simulink library "csu_lat_landing_approach_targeting_lib"  (R2014b)
settings: Solver=ode45  StartTime=0.0  StopTime=10.0  RelTol=1e-3
libraries: simulink x8, util_info_lib x1, util_common_lib x1
settings Model: Creator=escrane  LastModifiedBy=Mark Agbayani

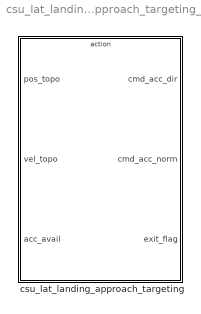
== system csu_lat_landing_approach_targeting_lib ==
  csu_lat_landing_approach_targeting : Subsystem  TreatAsAtomicUnit=on

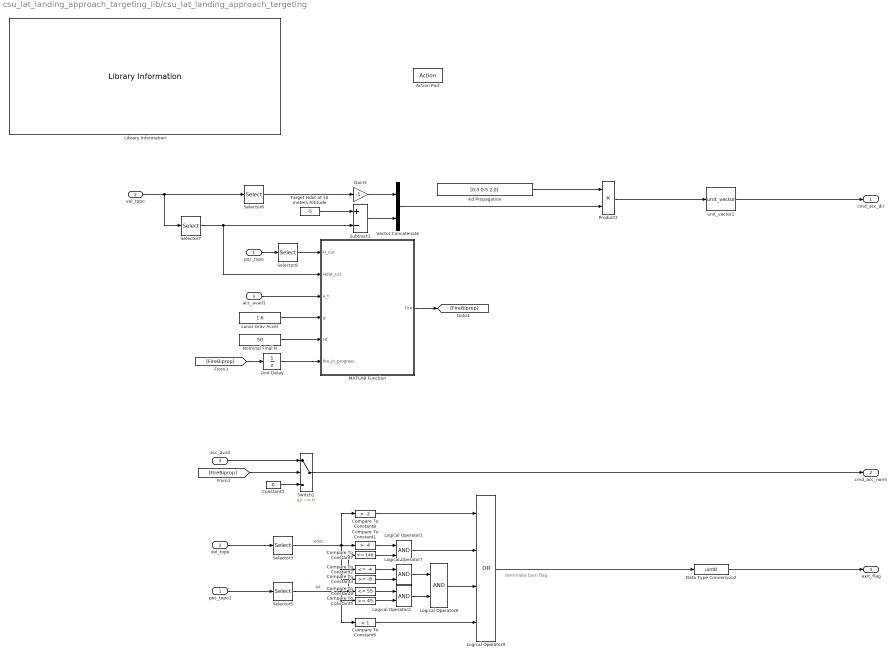
== system csu_lat_landing_approach_targeting_lib/csu_lat_landing_approach_targeting ==
  note: terminate burn flag
  "pos_topo " : Inport
  "vel_topo " : Inport  Port=2
  acc_avail : Inport  Port=3
  Action Port : ActionPort
  Compare To Constant1 : simulink/Logic and Bit Operations/Compare To Constant  relop=>  const=-4  OutDataTypeStr=boolean
  Compare To Constant2 : simulink/Logic and Bit Operations/Compare To Constant  relop=<=  const=-4  OutDataTypeStr=boolean
  Compare To Constant3 : simulink/Logic and Bit Operations/Compare To Constant  relop=>=  const=-8  OutDataTypeStr=boolean
  Compare To Constant4 : simulink/Logic and Bit Operations/Compare To Constant  relop=<=  const=55  OutDataTypeStr=boolean
  Compare To Constant5 : simulink/Logic and Bit Operations/Compare To Constant  relop=>=  const=45  OutDataTypeStr=boolean
  Compare To Constant6 : simulink/Logic and Bit Operations/Compare To Constant  relop=<  const=1  OutDataTypeStr=boolean
  Compare To Constant7 : simulink/Logic and Bit Operations/Compare To Constant  relop=<=  const=140  OutDataTypeStr=boolean
  Compare To Constant8 : simulink/Logic and Bit Operations/Compare To Constant  relop=>  const=-2  OutDataTypeStr=boolean
  Constant3 : Constant  Value=0
  Data Type Conversion2 : DataTypeConversion  OutDataTypeStr=uint8
  Gain5 : Gain  Gain=-1
  "Kd Propagation " : Constant  Value=[0.5 0.5 2.0]
  Library Information : util_info_lib/Library Information  owner='NONE'
  Logical Operator{1..2,7..8} (4 alike) : Logic  AllPortsSameDT=off  OutDataTypeStr=boolean
  Logical Operator9 : Logic  Operator=OR  Inputs=4  AllPortsSameDT=off  OutDataTypeStr=boolean
  Lunar Grav Accel : Constant  Value=1.6
  MATLAB Function : MATLAB Function  TreatAsAtomicUnit=on
  "Nominal Final H " : Constant  Value=50
  Product2 : Product
  Selector{3,5,7..8} (4 alike) : Selector  InputPortWidth=3  Indices=[3]
  Selector6 : Selector  InputPortWidth=3  Indices=[1 2]
  Subtract1 : Sum  Inputs=+-
  Switch1 : Switch  Criteria=u2 ~= 0
  Target Hdot at 50 meters Altitude : Constant  Value=-5
  Unit Delay : UnitDelay  SampleTime=-1
  Vector Concatenate : Concatenate
  acc_avail1 : InportShadow  Port=3
  pos_topo1 : InportShadow
  unit_vector1 : util_common_lib/unit_vector  SystemSampleTime=-1
  vel_topo : InportShadow  Port=2
  cmd_acc_dir : Outport  InitialOutput=[0 0 1]'
  cmd_acc_norm : Outport  Port=2  InitialOutput=0
  exit_flag : Outport  Port=3  InitialOutput=0
  wires:
  Logical Operator9/1 -> Data Type Conversion2/1
  Data Type Conversion2/1 -> exit_flag/1
  "vel_topo "/1 -> Selector7/1, Selector6/1
  Selector8/1 -> MATLAB Function/1(H_cur)
  Product2/1 -> unit_vector1/1
  unit_vector1/1 -> cmd_acc_dir/1
  Compare To Constant3/1 -> Logical Operator7/2
  Compare To Constant6/1 -> Logical Operator9/4
  Selector5/1 -> Compare To Constant7/1, Compare To Constant4/1, Compare To Constant5/1, Compare To Constant6/1  "Alt"
  Selector3/1 -> Compare To Constant8/1, Compare To Constant1/1, Compare To Constant2/1, Compare To Constant3/1  "Hdot"
  Compare To Constant2/1 -> Logical Operator7/1
  Logical Operator8/1 -> Logical Operator9/3
  pos_topo1/1 -> Selector5/1
  vel_topo/1 -> Selector3/1
  MATLAB Function/1(Fire) -> [FireBiprop]
  "pos_topo "/1 -> Selector8/1
  Vector Concatenate/1 -> Product2/2
  Subtract1/1 -> Vector Concatenate/2
  Gain5/1 -> Vector Concatenate/1
  Selector7/1 -> Subtract1/2, MATLAB Function/2(Hdot_cur)
  Target Hdot at 50 meters Altitude/1 -> Subtract1/1
  Selector6/1 -> Gain5/1
  "Kd Propagation "/1 -> Product2/1
  Switch1/1 -> cmd_acc_norm/1
  Constant3/1 -> Switch1/3
  [FireBiprop] -> Switch1/2
  Logical Operator7/1 -> Logical Operator8/1
  Logical Operator2/1 -> Logical Operator8/2
  acc_avail1/1 -> MATLAB Function/3(a_t)
  [FireBiprop] -> Unit Delay/1
  Unit Delay/1 -> MATLAB Function/6(fire_in_progress)
  "Nominal Final H "/1 -> MATLAB Function/5(Hf)
  Lunar Grav Accel/1 -> MATLAB Function/4(g)
  Compare To Constant4/1 -> Logical Operator2/1
  Compare To Constant5/1 -> Logical Operator2/2
  acc_avail/1 -> Switch1/1
  Compare To Constant1/1 -> Logical Operator1/1
  Compare To Constant7/1 -> Logical Operator1/2
  Logical Operator1/1 -> Logical Operator9/2
  Compare To Constant8/1 -> Logical Operator9/1

== matlab function csu_lat_landing_approach_targeting_lib/csu_lat_landing_approach_targeting/MATLAB Function ==
  data: H_cur input; Hdot_cur input; Fire output boolean; a_t input; g input; Hf input; fire_in_progress input boolean
function Fire = ApproachTargeting(H_cur,Hdot_cur,a_t,g,Hf,fire_in_progress)
%#codegen

Hi = H_cur;
Hdoti = Hdot_cur;

if fire_in_progress == 0
    
    if (Hdoti^2 - 2*(a_t - g)*(Hi - Hf)) >= 0
       tf = (-Hdoti + sqrt(Hdoti^2 - 2*(a_t - g)*(Hi - Hf)))/(a_t - g);
    else
      tf = -1;
    end

    if tf > 0; 
        Fire = true;
    else
        Fire = false;
    end
else   
    Fire = true;
end
